simulink model "sampleModel1643"  (R2023a)
settings: Solver=VariableStepAuto  StartTime=0.0  StopTime=10.0  RelTol=1e-3
libraries: hdlsllib x5
settings Model: Creator=user1  LastModifiedBy=user1

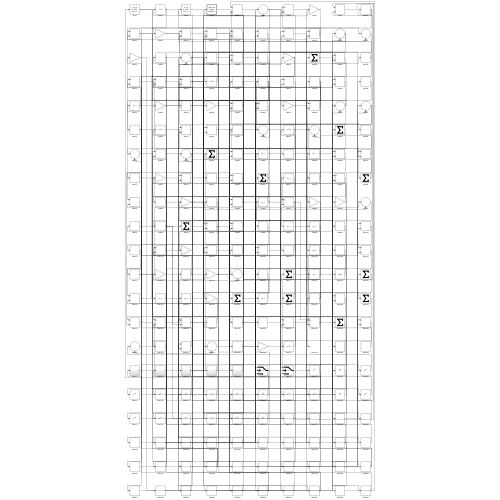
[thumbnail: Simulink's stored preview of the top-level diagram]
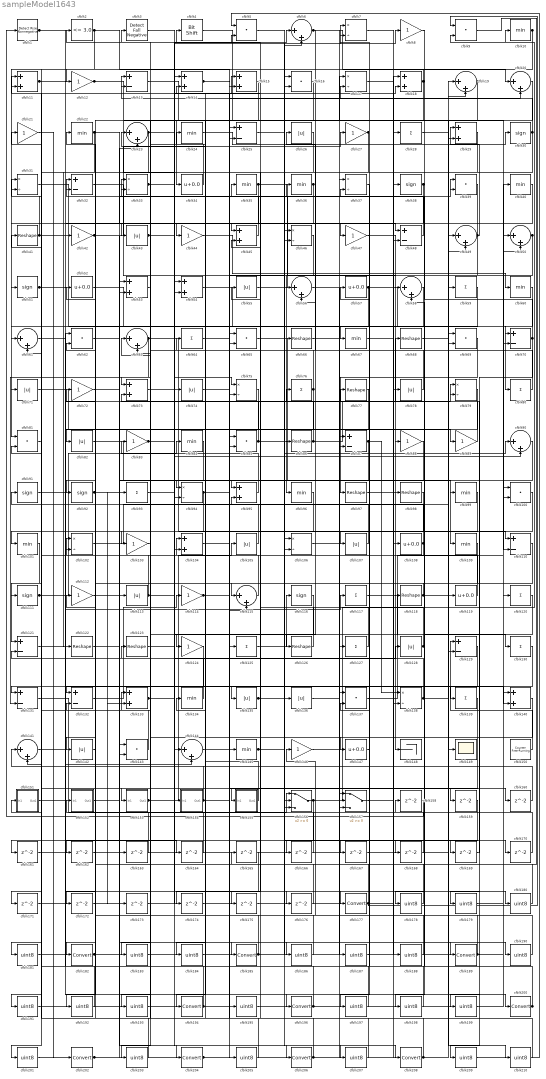
== system sampleModel1643 ==
  cfblk1 : hdlsllib/Logic and Bit Operations/Detect Rise Nonnegative  vinit=0  OutDataTypeStr=boolean
  cfblk{10,22,24,35..36,40,60,67,84,96,99,101,109,134,145} (15 alike) : MinMax
  cfblk{5,9,16,39,62,65,69,81,85,100,137,143} (12 alike) : DotProduct  OutDataTypeStr=Inherit: Inherit via internal rule
  cfblk{7,17,31,33,37,46,75,79,94,102,106,138} (12 alike) : Product  Inputs=*/  RndMeth=Zero  SaturateOnIntegerOverflow=on
  cfblk{8,12,21,27,42,44,47,72,83,88..89,103,112,114,124,146} (16 alike) : Gain
  cfblk{11,14..15,18,29,45,53..54,73,95,104,133,140} (13 alike) : Sum
  cfblk{26,43,55,71,74,78,82,105,107,113,128,135..136,142} (14 alike) : Abs  SaturateOnIntegerOverflow=off
  cfblk{34,52,57,108,119,147} (6 alike) : Bias  Bias=0.0  SaturateOnIntegerOverflow=off
  cfblk{13,25,32,48,70,87,110,121,129,131..132} (11 alike) : Sum  Inputs=+-
  cfblk{30,38,51,91..92,111,116} (7 alike) : Signum
  cfblk{6,19..20,23,49..50,56,58,61,63,90,115,141,144} (14 alike) : Sum  Inputs=|++
  cfblk{28,59,64,76,80,93,117,120,125,127,130,139} (12 alike) : Sum  Inputs=+
  cfblk{41,66,68,77,86,97..98,118,122..123,126} (11 alike) : Reshape
  cfblk148 : Terminator
  cfblk149 : Scope
  cfblk150 : hdlsllib/Sources/Counter Free-Running  NumBits=16  tsamp=-1
  cfblk151 : Subsystem
      settings: LibrarySourceBlock=|
      | hdlsllib/Ports &
      | Subsystems/Subsystem
  cfblk152 : Subsystem
      settings: LibrarySourceBlock=|
      | hdlsllib/Ports &
      | Subsystems/Subsystem
  cfblk153 : Subsystem
      settings: LibrarySourceBlock=|
      | hdlsllib/Ports &
      | Subsystems/Subsystem
  cfblk154 : Subsystem
      settings: LibrarySourceBlock=|
      | hdlsllib/Ports &
      | Subsystems/Subsystem
  cfblk155 : Subsystem
      settings: LibrarySourceBlock=|
      | hdlsllib/Ports &
      | Subsystems/Subsystem
  cfblk156 : Switch  SaturateOnIntegerOverflow=off  InputSameDT=off
  cfblk157 : Switch  SaturateOnIntegerOverflow=off  InputSameDT=off
  cfblk{158..176} (19 alike) : Delay  SampleTime=1
  cfblk{177,182,185,189,194,196,200,202,204,206,208} (11 alike) : DataTypeConversion  SaturateOnIntegerOverflow=off  RndMeth=Floor
  cfblk{178..181,183..184,186..188,190..193,195,197..199,201,203,205,207,209..210} (23 alike) : DataTypeConversion  OutDataTypeStr=uint8  SaturateOnIntegerOverflow=off  RndMeth=Floor
  cfblk2 : hdlsllib/Logic and Bit Operations/Compare To Constant  relop=<=  const=3.0  OutDataTypeStr=boolean
  cfblk3 : hdlsllib/Logic and Bit Operations/Detect Fall Negative  vinit=0  OutDataTypeStr=boolean
  cfblk4 : hdlsllib/Logic and Bit Operations/Bit Shift  mode=Shift Left Logical  N=0
  wires:
  cfblk54/1 -> cfblk67/1
  cfblk112/1 -> cfblk204/1
  cfblk63/1 -> cfblk107/1, cfblk131/2
  cfblk22/1 -> cfblk122/1, cfblk48/2
  cfblk44/1 -> cfblk60/1
  cfblk2/1 -> cfblk81/1, cfblk15/2
  cfblk118/1 -> cfblk115/1, cfblk210/1
  cfblk111/1 -> cfblk84/1, cfblk144/2
  cfblk99/1 -> cfblk104/1
  cfblk42/1 -> cfblk27/1, cfblk95/1
  cfblk69/1 -> cfblk97/1
  cfblk153/1(Out1) -> cfblk105/1, cfblk39/2, cfblk128/1
  cfblk126/1 -> cfblk2/1
  cfblk131/1 -> cfblk156/1
  cfblk19/1 -> cfblk124/1, cfblk17/2
  cfblk34/1 -> cfblk11/1
  cfblk49/1 -> cfblk44/1, cfblk29/1, cfblk75/2
  cfblk18/1 -> cfblk12/1, cfblk56/1
  cfblk156/1 -> cfblk10/1, cfblk166/1
  cfblk151/1(Out1) -> cfblk196/1
  cfblk127/1 -> cfblk4/1
  cfblk36/1 -> cfblk51/1, cfblk101/1, cfblk43/1
  cfblk31/1 -> cfblk96/1
  cfblk130/1 -> cfblk132/1
  cfblk30/1 -> cfblk135/1, cfblk13/2
  cfblk29/1 -> cfblk73/1
  cfblk121/1 -> cfblk77/1
  cfblk4/1 -> cfblk149/1
  cfblk82/1 -> cfblk109/1
  cfblk108/1 -> cfblk91/1, cfblk102/2
  cfblk65/1 -> cfblk127/1
  cfblk3/1 -> cfblk177/1
  cfblk115/1 -> cfblk102/1
  cfblk76/1 -> cfblk82/1, cfblk55/1
  cfblk94/1 -> cfblk125/1, cfblk111/1
  cfblk98/1 -> cfblk104/2
  cfblk60/1 -> cfblk80/1
  cfblk16/1 -> cfblk182/1
  cfblk66/1 -> cfblk89/1
  cfblk52/1 -> cfblk154/1(In1)
  cfblk132/1 -> cfblk114/1
  cfblk47/1 -> cfblk148/1
  cfblk38/1 -> cfblk155/1(In1), cfblk118/1, cfblk147/1
  cfblk86/1 -> cfblk68/1, cfblk45/2
  cfblk40/1 -> cfblk194/1
  cfblk89/1 -> cfblk73/2
  cfblk20/1 -> cfblk34/1
  cfblk110/1 -> cfblk142/1
  cfblk68/1 -> cfblk49/1
  cfblk45/1 -> cfblk24/1
  cfblk24/1 -> cfblk30/1
  cfblk39/1 -> cfblk47/1
  cfblk55/1 -> cfblk39/1
  cfblk97/1 -> cfblk28/1
  cfblk58/1 -> cfblk131/1
  cfblk7/1 -> cfblk108/1
  cfblk117/1 -> cfblk130/1
  cfblk150/1 -> cfblk129/1
  cfblk23/1 -> cfblk87/1, cfblk75/1, cfblk92/1
  cfblk84/1 -> cfblk143/2
  cfblk32/1 -> cfblk136/1
  cfblk5/1 -> cfblk208/1
  cfblk41/1 -> cfblk42/1, cfblk31/1
  cfblk107/1 -> cfblk64/1
  cfblk26/1 -> cfblk71/1
  cfblk119/1 -> cfblk11/2
  cfblk129/1 -> cfblk156/2
  cfblk135/1 -> cfblk90/1, cfblk167/1
  cfblk87/1 -> cfblk106/2, cfblk138/1
  cfblk92/1 -> cfblk37/2, cfblk133/2, cfblk173/1
  cfblk101/1 -> cfblk121/1
  cfblk11/1 -> cfblk45/1, cfblk138/2
  cfblk57/1 -> cfblk119/1, cfblk94/2
  cfblk95/1 -> cfblk83/1
  cfblk72/1 -> cfblk185/1
  cfblk105/1 -> cfblk33/1
  cfblk79/1 -> cfblk94/1
  cfblk145/1 -> cfblk7/1, cfblk169/1
  cfblk83/1 -> cfblk8/1, cfblk176/1
  cfblk141/1 -> cfblk117/1
  cfblk71/1 -> cfblk144/1
  cfblk134/1 -> cfblk81/2
  cfblk43/1 -> cfblk48/1, cfblk70/1
  cfblk14/1 -> cfblk139/1, cfblk160/1
  cfblk103/1 -> cfblk63/2
  cfblk6/1 -> cfblk20/1, cfblk29/2, cfblk126/1
  cfblk113/1 -> cfblk129/2, cfblk41/1
  cfblk102/1 -> cfblk69/2
  cfblk136/1 -> cfblk87/2
  cfblk128/1 -> cfblk57/1, cfblk13/1
  cfblk35/1 -> cfblk58/1, cfblk174/1
  cfblk133/1 -> cfblk6/1, cfblk207/1
  cfblk33/1 -> cfblk99/1, cfblk90/2, cfblk70/2
  cfblk13/1 -> cfblk145/1
  cfblk50/1 -> cfblk156/3, cfblk56/2
  cfblk106/1 -> cfblk79/1
  cfblk53/1 -> cfblk153/1(In1)
  cfblk21/1 -> cfblk202/1
  cfblk138/1 -> cfblk31/2, cfblk170/1
  cfblk137/1 -> cfblk50/2
  cfblk85/1 -> cfblk157/1, cfblk14/2
  cfblk67/1 -> cfblk38/1
  cfblk125/1 -> cfblk116/1
  cfblk46/1 -> cfblk86/1
  cfblk12/1 -> cfblk74/1, cfblk110/2
  cfblk90/1 -> cfblk157/2
  cfblk114/1 -> cfblk115/2, cfblk18/2
  cfblk80/1 -> cfblk36/1
  cfblk25/1 -> cfblk189/1
  cfblk51/1 -> cfblk88/1, cfblk61/2
  cfblk70/1 -> cfblk32/1, cfblk199/1
  cfblk144/1 -> cfblk20/2
  cfblk155/1(Out1) -> cfblk23/1
  cfblk93/1 -> cfblk200/1
  cfblk62/1 -> cfblk53/2
  cfblk104/1 -> cfblk110/1
  cfblk154/1(Out1) -> cfblk76/1, cfblk133/1
  cfblk123/1 -> cfblk206/1
  cfblk27/1 -> cfblk54/2, cfblk181/1
  cfblk15/1 -> cfblk103/1
  cfblk147/1 -> cfblk7/2
  cfblk48/1 -> cfblk26/1
  cfblk152/1(Out1) -> cfblk113/1
  cfblk77/1 -> cfblk85/2
  cfblk124/1 -> cfblk141/2
  cfblk10/1 -> cfblk61/1, cfblk9/2
  cfblk78/1 -> cfblk32/2
  cfblk143/1 -> cfblk121/2
  cfblk73/1 -> cfblk15/1
  cfblk1/1 -> cfblk46/2, cfblk140/2
  cfblk158/1 -> cfblk1/1
  cfblk157/1 -> cfblk159/1
  cfblk160/1 -> cfblk141/1
  cfblk139/1 -> cfblk161/1
  cfblk161/1 -> cfblk14/1
  cfblk142/1 -> cfblk162/1
  cfblk162/1 -> cfblk19/1
  cfblk163/1 -> cfblk53/1
  cfblk61/1 -> cfblk164/1
  cfblk164/1 -> cfblk63/1
  cfblk9/1 -> cfblk165/1
  cfblk166/1 -> cfblk33/2
  cfblk167/1 -> cfblk49/2
  cfblk56/1 -> cfblk168/1
  cfblk168/1 -> cfblk46/1
  cfblk169/1 -> cfblk79/2
  cfblk170/1 -> cfblk132/2
  cfblk96/1 -> cfblk171/1
  cfblk171/1 -> cfblk106/1
  cfblk75/1 -> cfblk172/1
  cfblk172/1 -> cfblk23/2
  cfblk173/1 -> cfblk54/1
  cfblk174/1 -> cfblk37/1
  cfblk109/1 -> cfblk175/1
  cfblk175/1 -> cfblk18/1
  cfblk176/1 -> cfblk95/2
  cfblk177/1 -> cfblk9/1, cfblk52/1
  cfblk8/1 -> cfblk178/1
  cfblk178/1 -> cfblk3/1
  cfblk100/1 -> cfblk179/1
  cfblk179/1 -> cfblk50/1
  cfblk91/1 -> cfblk180/1
  cfblk180/1 -> cfblk100/1
  cfblk181/1 -> cfblk100/2
  cfblk182/1 -> cfblk163/1, cfblk66/1, cfblk65/2
  cfblk116/1 -> cfblk183/1
  cfblk183/1 -> cfblk16/1
  cfblk165/1 -> cfblk184/1
  cfblk184/1 -> cfblk16/2
  cfblk185/1 -> cfblk6/2, cfblk152/1(In1)
  cfblk122/1 -> cfblk186/1
  cfblk186/1 -> cfblk72/1
  cfblk146/1 -> cfblk187/1
  cfblk187/1 -> cfblk98/1
  cfblk17/1 -> cfblk188/1
  cfblk188/1 -> cfblk146/1
  cfblk189/1 -> cfblk158/1, cfblk209/1
  cfblk28/1 -> cfblk190/1
  cfblk190/1 -> cfblk25/1
  cfblk159/1 -> cfblk191/1
  cfblk191/1 -> cfblk25/2
  cfblk59/1 -> cfblk192/1
  cfblk192/1 -> cfblk62/1
  cfblk140/1 -> cfblk193/1
  cfblk193/1 -> cfblk59/1
  cfblk194/1 -> cfblk22/1, cfblk62/2, cfblk143/1
  cfblk74/1 -> cfblk195/1
  cfblk195/1 -> cfblk40/1
  cfblk196/1 -> cfblk140/1, cfblk35/1
  cfblk37/1 -> cfblk197/1
  cfblk197/1 -> cfblk151/1(In1)
  cfblk120/1 -> cfblk198/1
  cfblk198/1 -> cfblk137/2
  cfblk199/1 -> cfblk120/1
  cfblk200/1 -> cfblk58/2, cfblk137/1
  cfblk81/1 -> cfblk201/1
  cfblk201/1 -> cfblk93/1
  cfblk202/1 -> cfblk78/1, cfblk19/2
  cfblk88/1 -> cfblk203/1
  cfblk203/1 -> cfblk21/1
  cfblk204/1 -> cfblk157/3, cfblk69/1
  cfblk64/1 -> cfblk205/1
  cfblk205/1 -> cfblk112/1
  cfblk206/1 -> cfblk134/1, cfblk65/1
  cfblk207/1 -> cfblk123/1
  cfblk208/1 -> cfblk17/1, cfblk85/1
  cfblk209/1 -> cfblk5/1
  cfblk210/1 -> cfblk5/2

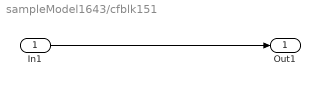
== system sampleModel1643/cfblk151 ==
  In1 : Inport
  Out1 : Outport
  wires:
  In1/1 -> Out1/1

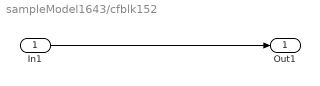
== system sampleModel1643/cfblk152 ==
  In1 : Inport
  Out1 : Outport
  wires:
  In1/1 -> Out1/1

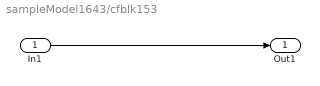
== system sampleModel1643/cfblk153 ==
  In1 : Inport
  Out1 : Outport
  wires:
  In1/1 -> Out1/1

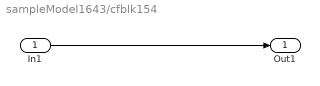
== system sampleModel1643/cfblk154 ==
  In1 : Inport
  Out1 : Outport
  wires:
  In1/1 -> Out1/1

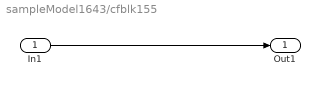
== system sampleModel1643/cfblk155 ==
  In1 : Inport
  Out1 : Outport
  wires:
  In1/1 -> Out1/1
